simulink library "csu_spv_simulated_press_valves_lib"  (R2014b)
settings: Solver=ode45  StartTime=0.0  StopTime=10.0  RelTol=1e-3
values from neighbouring files (symbols this model uses):
  sim_time_step_size = 0.01    [csu_tdl_thruster_dynamics_lander_test.m]    (also in sim_thruster_wsim_test.m)
undefined symbols (not defined in the file or in its folder): tdl_valve_delay_cycles
libraries: simulink x1, util_info_lib x1
settings Model: Creator=Nilesh  LastModifiedBy=mstewart

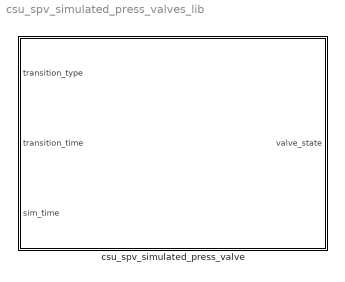
== system csu_spv_simulated_press_valves_lib ==
  csu_spv_simulated_press_valve : Subsystem  mask{thruster_idx=[], num_thrusters=[], energized_value=[], deenergized_value=[]}
      mask prompts: thruster_idx "Thruster Index (1-total)"; num_thrusters "Number of thrusters (total)"; energized_value "Energized State (closed = 0, open = 1)"; deenergized_value "De-energized State (closed = 0, open = 1)"

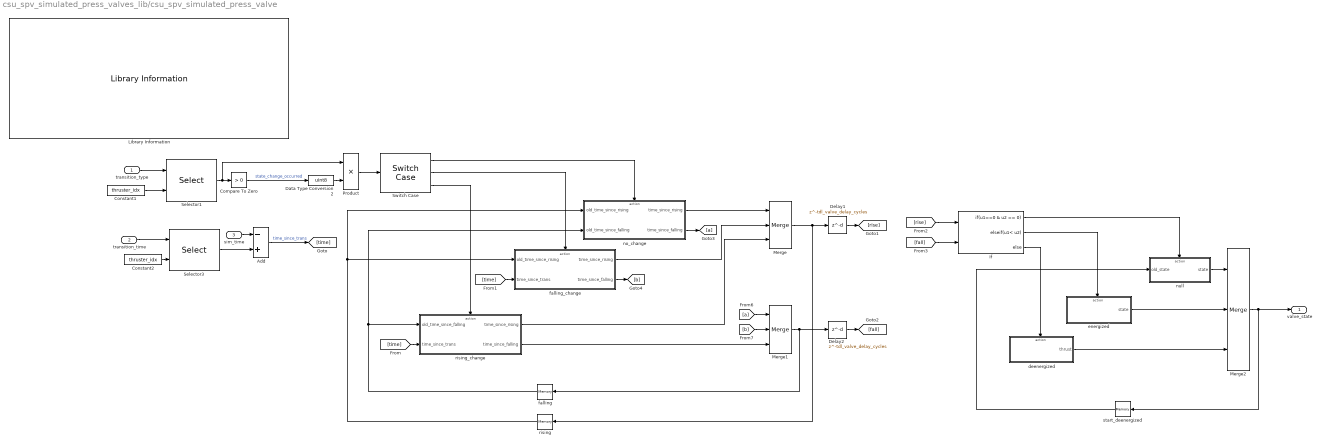
== system csu_spv_simulated_press_valves_lib/csu_spv_simulated_press_valve ==
  transition_type : Inport
  transition_time : Inport  Port=2
  sim_time : Inport  Port=3
  Add : Sum  Inputs=-+
  Compare To Zero : simulink/Logic and Bit Operations/Compare To Zero  relop=>  OutDataTypeStr=boolean
  Constant1 : Constant  Value=thruster_idx  OutDataTypeStr=uint8
  Constant2 : Constant  Value=thruster_idx  OutDataTypeStr=uint8
  Data Type Conversion2 : DataTypeConversion  OutDataTypeStr=uint8
  Delay1 : Delay  DelayLength=tdl_valve_delay_cycles
  Delay2 : Delay  DelayLength=tdl_valve_delay_cycles
  If : If  NumInputs=2  IfExpression=u1==0 & u2 == 0  ElseIfExpressions=u1< u2
  Library Information : util_info_lib/Library Information  owner='escrane'
  Merge : Merge  Inputs=3
  Merge1 : Merge  Inputs=3
  Merge2 : Merge  Inputs=3
  Product : Product
  Selector1 : Selector  InputPortWidth=num_thrusters  IndexOptions=Index vector (port)  Indices=[1 3]
  Selector3 : Selector  InputPortWidth=num_thrusters  IndexOptions=Index vector (port)  Indices=[1 3]
  Switch Case : SwitchCase  CaseConditions={0,1,2}  ShowDefaultCase=off
  deenergized : Subsystem  TreatAsAtomicUnit=on
  energized : Subsystem  TreatAsAtomicUnit=on
  falling : Memory  InheritSampleTime=on
  falling_change : Subsystem  TreatAsAtomicUnit=on
  no_change : Subsystem  TreatAsAtomicUnit=on
  null : Subsystem  TreatAsAtomicUnit=on
  rising : Memory  InheritSampleTime=on
  rising_change : Subsystem  TreatAsAtomicUnit=on
  start_deenergized : Memory  X0=uint8(deenergized_value)  InheritSampleTime=on
  valve_state : Outport
  wires:
  If/1 -> null/Action
  null/1(state) -> Merge2/1
  energized/1(state) -> Merge2/2
  deenergized/1(thrust) -> Merge2/3
  If/2 -> energized/Action
  Delay2/1 -> [fall]
  Delay1/1 -> [rise]
  Merge1/1 -> falling/1, Delay2/1
  Merge/1 -> rising/1, Delay1/1
  [b] -> Merge1/2
  falling_change/2(time_since_falling) -> [b]
  [a] -> Merge1/1
  no_change/2(time_since_falling) -> [a]
  no_change/1(time_since_rising) -> Merge/1
  If/3 -> deenergized/Action
  [rise] -> If/1
  [fall] -> If/2
  sim_time/1 -> Add/1
  Compare To Zero/1 -> Data Type Conversion2/1  "state_change_occurred"
  Data Type Conversion2/1 -> Product/2
  Add/1 -> [time]  "time_since_trans"
  Product/1 -> Switch Case/1
  Switch Case/1 -> no_change/Action
  Switch Case/2 -> falling_change/Action
  Switch Case/3 -> rising_change/Action
  [time] -> rising_change/2(time_since_trans)
  [time] -> falling_change/2(time_since_trans)
  falling/1 -> rising_change/1(old_time_since_falling), no_change/2(old_time_since_falling)
  rising/1 -> falling_change/1(old_time_since_rising), no_change/1(old_time_since_rising)
  falling_change/1(time_since_rising) -> Merge/2
  rising_change/1(time_since_rising) -> Merge/3
  rising_change/2(time_since_falling) -> Merge1/3
  Constant2/1 -> Selector3/2
  transition_time/1 -> Selector3/1
  Selector3/1 -> Add/2
  Constant1/1 -> Selector1/2
  transition_type/1 -> Selector1/1
  Selector1/1 -> Product/1, Compare To Zero/1
  start_deenergized/1 -> null/1(old_state)
  Merge2/1 -> start_deenergized/1, valve_state/1

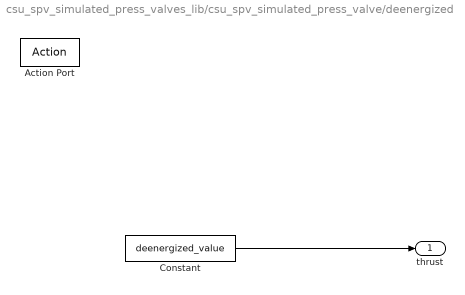
== system csu_spv_simulated_press_valves_lib/csu_spv_simulated_press_valve/deenergized ==
  Action Port : ActionPort
  Constant : Constant  Value=deenergized_value  OutDataTypeStr=uint8
  thrust : Outport  InitialOutput=0
  wires:
  Constant/1 -> thrust/1

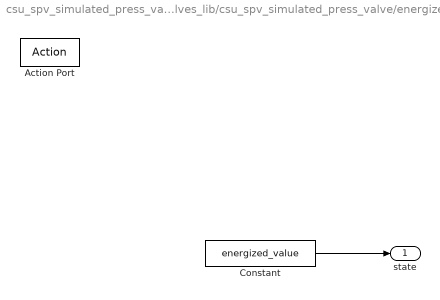
== system csu_spv_simulated_press_valves_lib/csu_spv_simulated_press_valve/energized ==
  Action Port : ActionPort
  Constant : Constant  Value=energized_value  OutDataTypeStr=uint8
  state : Outport  InitialOutput=0
  wires:
  Constant/1 -> state/1

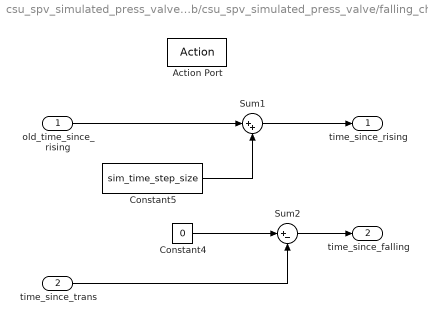
== system csu_spv_simulated_press_valves_lib/csu_spv_simulated_press_valve/falling_change ==
  old_time_since_rising : Inport
  time_since_trans : Inport  Port=2
  Action Port : ActionPort
  Constant4 : Constant  Value=0
  Constant5 : Constant  Value=sim_time_step_size
  Sum1 : Sum  Inputs=|++
  Sum2 : Sum  Inputs=|+-
  time_since_rising : Outport
  time_since_falling : Outport  Port=2
  wires:
  Constant4/1 -> Sum2/1
  Sum1/1 -> time_since_rising/1
  old_time_since_rising/1 -> Sum1/1
  Constant5/1 -> Sum1/2
  time_since_trans/1 -> Sum2/2
  Sum2/1 -> time_since_falling/1

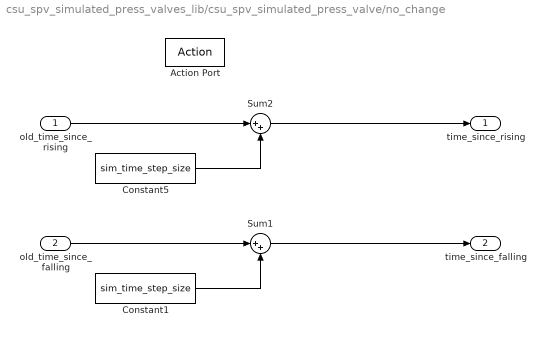
== system csu_spv_simulated_press_valves_lib/csu_spv_simulated_press_valve/no_change ==
  old_time_since_rising : Inport
  old_time_since_falling : Inport  Port=2
  Action Port : ActionPort
  Constant1 : Constant  Value=sim_time_step_size
  Constant5 : Constant  Value=sim_time_step_size
  Sum1 : Sum  Inputs=|++
  Sum2 : Sum  Inputs=|++
  time_since_rising : Outport
  time_since_falling : Outport  Port=2
  wires:
  old_time_since_rising/1 -> Sum2/1
  Constant5/1 -> Sum2/2
  Sum2/1 -> time_since_rising/1
  old_time_since_falling/1 -> Sum1/1
  Constant1/1 -> Sum1/2
  Sum1/1 -> time_since_falling/1

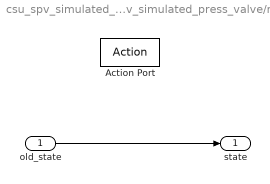
== system csu_spv_simulated_press_valves_lib/csu_spv_simulated_press_valve/null ==
  old_state : Inport
  Action Port : ActionPort
  state : Outport  InitialOutput=0
  wires:
  old_state/1 -> state/1

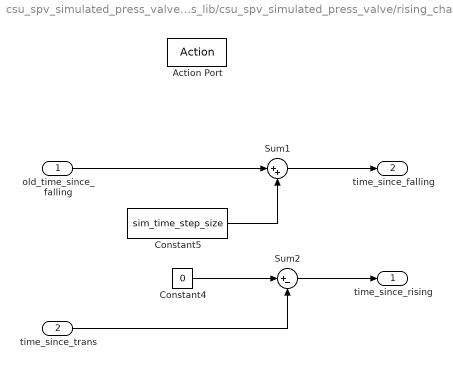
== system csu_spv_simulated_press_valves_lib/csu_spv_simulated_press_valve/rising_change ==
  old_time_since_falling : Inport
  time_since_trans : Inport  Port=2
  Action Port : ActionPort
  Constant4 : Constant  Value=0
  Constant5 : Constant  Value=sim_time_step_size
  Sum1 : Sum  Inputs=|++
  Sum2 : Sum  Inputs=|+-
  time_since_rising : Outport
  time_since_falling : Outport  Port=2
  wires:
  Sum2/1 -> time_since_rising/1
  Constant4/1 -> Sum2/1
  time_since_trans/1 -> Sum2/2
  old_time_since_falling/1 -> Sum1/1
  Sum1/1 -> time_since_falling/1
  Constant5/1 -> Sum1/2
